simulink model "sample"  (R2018b)
settings: Solver=FixedStepDiscrete  StartTime=0.0  StopTime=10.0  RelTol=1e-3
settings Model: Creator=a_miyazaki  LastModifiedBy=a_miyazaki

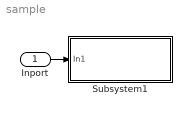
== system sample ==
  Inport : Inport
  Subsystem1 : Subsystem
  wires:
  Inport/1 -> Subsystem1/1(In1)

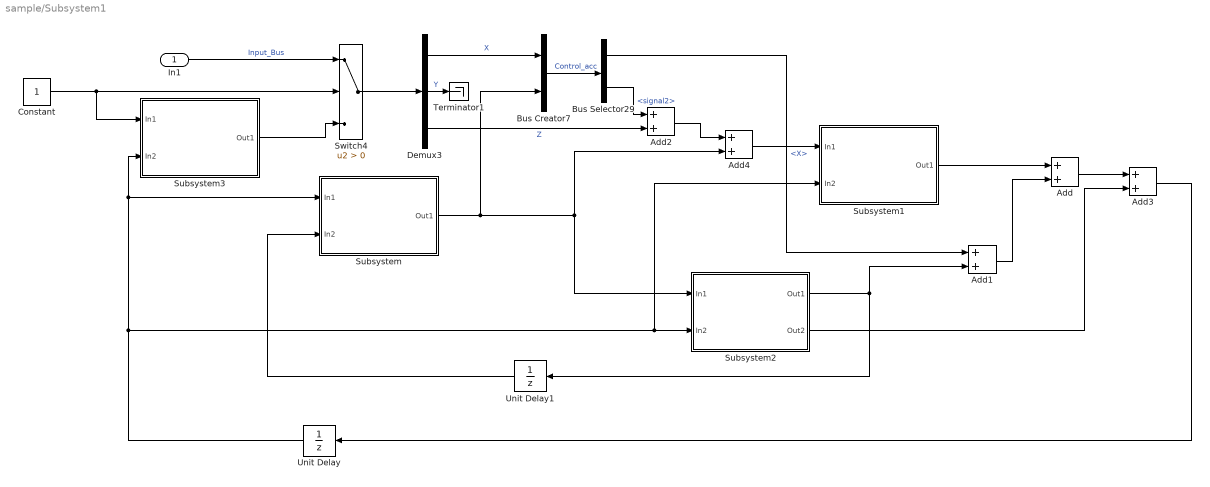
== system sample/Subsystem1 ==
  In1 : Inport
  Add{,1..4} (5 alike) : Sum
  Bus Creator7 : BusCreator  Inputs=2
  Bus Selector29 : BusSelector  OutputSignals=X,signal2
  Constant : Constant  SampleTime=-1
  Demux3 : Demux  Outputs=3
  Subsystem : Subsystem
  Subsystem1 : Subsystem
  Subsystem2 : Subsystem
  Subsystem3 : Subsystem
  Switch4 : Switch  Criteria=u2 > Threshold
  Terminator1 : Terminator
  Unit Delay : UnitDelay  SampleTime=-1
  Unit Delay1 : UnitDelay  SampleTime=-1
  wires:
  Subsystem2/2(Out2) -> Add3/2
  Subsystem1/1(Out1) -> Add/1
  Subsystem2/1(Out1) -> Unit Delay1/1, Add1/2
  Add1/1 -> Add/2
  In1/1 -> Switch4/1  "Input_Bus"
  Switch4/1 -> Demux3/1
  Demux3/1 -> Bus Creator7/1  "X"
  Bus Creator7/1 -> Bus Selector29/1  "Control_acc"
  Bus Selector29/1 -> Add1/1  "<X>"
  Demux3/3 -> Add2/2  "Z"
  Bus Selector29/2 -> Add2/1  "<signal2>"
  Add3/1 -> Unit Delay/1
  Add2/1 -> Add4/1
  Subsystem/1(Out1) -> Add4/2, Subsystem2/1(In1), Bus Creator7/2
  Demux3/2 -> Terminator1/1  "Y"
  Add4/1 -> Subsystem1/1(In1)
  Add/1 -> Add3/1
  Subsystem3/1(Out1) -> Switch4/3
  Constant/1 -> Subsystem3/1(In1), Switch4/2
  Unit Delay1/1 -> Subsystem/2(In2)
  Unit Delay/1 -> Subsystem/1(In1), Subsystem3/2(In2), Subsystem1/2(In2), Subsystem2/2(In2)

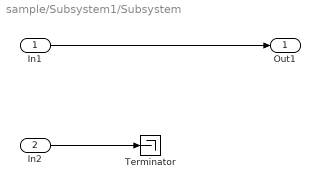
== system sample/Subsystem1/Subsystem ==
  In1 : Inport
  In2 : Inport  Port=2
  Terminator : Terminator
  Out1 : Outport
  wires:
  In1/1 -> Out1/1
  In2/1 -> Terminator/1

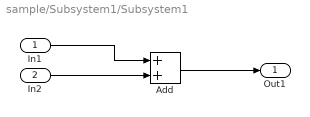
== system sample/Subsystem1/Subsystem1 ==
  In1 : Inport
  In2 : Inport  Port=2
  Add : Sum
  Out1 : Outport
  wires:
  In1/1 -> Add/1
  In2/1 -> Add/2
  Add/1 -> Out1/1

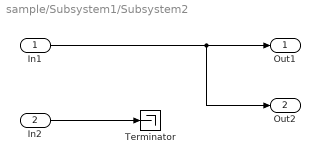
== system sample/Subsystem1/Subsystem2 ==
  In1 : Inport
  In2 : Inport  Port=2
  Terminator : Terminator
  Out1 : Outport
  Out2 : Outport  Port=2
  wires:
  In1/1 -> Out2/1, Out1/1
  In2/1 -> Terminator/1

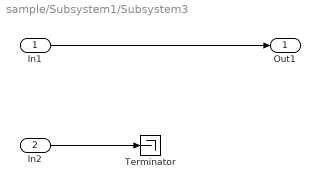
== system sample/Subsystem1/Subsystem3 ==
  In1 : Inport
  In2 : Inport  Port=2
  Terminator : Terminator
  Out1 : Outport
  wires:
  In1/1 -> Out1/1
  In2/1 -> Terminator/1
